simulink model "Vent_prop_valve_tuner"  (R2024b)
settings: Solver=ode15s  StartTime=0.0  StopTime=300  RelTol=1e-3
settings Model: Creator=MW  LastModifiedBy=MW

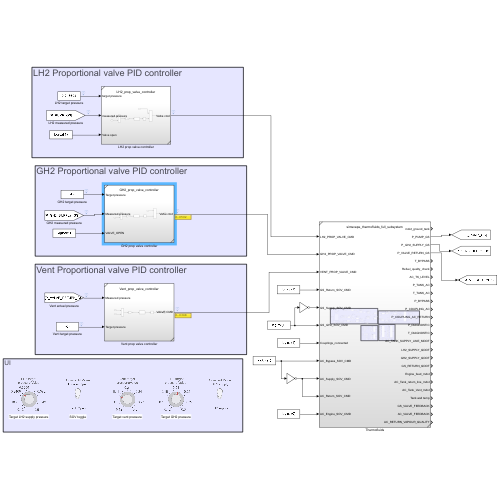
[thumbnail: Simulink's stored preview of the top-level diagram]
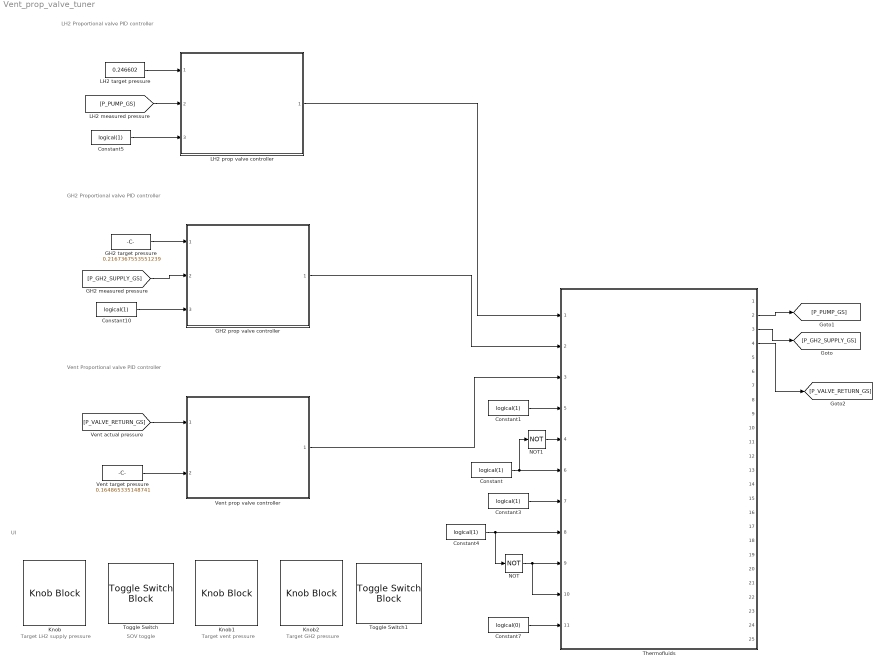
== system Vent_prop_valve_tuner ==
  note: Target LH2 supply pressure
  note: UI
  note: GH2 Proportional valve PID controller
  note: Target vent pressure
  note: SOV toggle
  note: LH2 Proportional valve PID controller
  note: Vent Proportional valve PID controller
  note: Target GH2 pressure
  Constant{,1,3..5,10} (6 alike) : Constant  Value=logical(1)
  Constant7 : Constant  Value=logical(0)
  GH2 prop valve controller : Subsystem  ReferencedSubsystem=GH2_prop_valve_controller
  GH2 target pressure : Constant  Value=0.2167367553551239
  Knob : KnobBlock  ScaleMin=0.12  ScaleMax=0.5
  Knob1 : KnobBlock  ScaleMin=0.12  ScaleMax=0.3
  Knob2 : KnobBlock  ScaleMin=0.12  ScaleMax=0.3
  LH2 prop valve controller : Subsystem  ReferencedSubsystem=LH2_prop_valve_controller
  LH2 target pressure : Constant  Value=0.246602
  NOT : Logic  Operator=NOT  IconShape=distinctive  AllPortsSameDT=off  OutDataTypeStr=boolean
  NOT1 : Logic  Operator=NOT  IconShape=distinctive  AllPortsSameDT=off  OutDataTypeStr=boolean
  Thermofluids : Subsystem  ReferencedSubsystem=simscape_thermofluids_full_subsystem
      settings: PortSchema="{\"entries\":[{\"content\":{\"sides\":[{\"content\":{\"connectorIds\":[\"In1\",\"In2\",\"In3\",\"In5\",\"In4\",\"In6\",\"In7\",\"In8\",\"In9\",\"In10\",\"In11\"]},\"type\":\"ConnectorPlacement.EquallySpacedRectSide\",\"uuid\":\"0abe1c09-fd1c-4f21-adb2-1ba1f178e40f\"},{\"content\":{\"connectorIds\":[\"Out1\",\"Out2\",\"Out3\",\"Out4\",\"Out5\",\"Out6\",\"Out7\",\"Out8\",\"Out9\",\"Out10\",\"Out11\",\"Out12\",\"Out13\",\"Out14\",\"Out15\",\"Out16\",\"Out17\",\"Out18\",\"Out19\",\"Out20\",\"Out21\",\"Out22\",\"Out23\",\"Out24\",\"Out25\"],\"side\":\"RIGHT\"},\"type\":\"ConnectorPlacement.EquallySpacedRectSide\",\"uuid\":\"d1a7e852-e313-42b4-9b52-713a379b8745\"},{\"content\":{\"side\":\"TOP\"},\"type\":\"ConnectorPlacement.EquallySpacedRectSide\",\"uuid\":\"bcf0416b-035c-45e3-b36d-7b1188a80ffd\"}]},\"type\":\"ConnectorPlacement.EquallySpacedConnector\",\"uuid\":\"eb213e55-2670-4e0e-a421-e9d6b5e6eb19\"}],\"packageUris\":[\"http://schema.mathworks.com/mf0/Connector/R2020b\"],\"version\":\"1.0\"}"
  Toggle Switch : ToggleSwitchBlock
      settings: Values={{'Tank Open', 'Bypass Open'}, [0 1]}
  Toggle Switch1 : ToggleSwitchBlock
      settings: Values={{'LH2 supply', 'GH2 supply'}, [0 1]}
  Vent prop valve controller : Subsystem  ReferencedSubsystem=Vent_prop_valve_controller
  Vent target pressure : Constant  Value=0.164865335148741
  wires:
  Constant1/1 -> Thermofluids/5
  Constant3/1 -> Thermofluids/7
  Constant4/1 -> NOT/1, Thermofluids/8
  NOT/1 -> Thermofluids/9, Thermofluids/10
  Constant7/1 -> Thermofluids/11
  GH2 target pressure/1 -> GH2 prop valve controller/1
  Constant10/1 -> GH2 prop valve controller/3
  [P_GH2_SUPPLY_GS] -> GH2 prop valve controller/2
  Thermofluids/3 -> [P_GH2_SUPPLY_GS]
  LH2 prop valve controller/1 -> Thermofluids/1
  GH2 prop valve controller/1 -> Thermofluids/2
  LH2 target pressure/1 -> LH2 prop valve controller/1
  [P_PUMP_GS] -> LH2 prop valve controller/2
  Constant5/1 -> LH2 prop valve controller/3
  Thermofluids/2 -> [P_PUMP_GS]
  Vent prop valve controller/1 -> Thermofluids/3
  Vent target pressure/1 -> Vent prop valve controller/2
  Thermofluids/4 -> [P_VALVE_RETURN_GS]
  [P_VALVE_RETURN_GS] -> Vent prop valve controller/1
  NOT1/1 -> Thermofluids/4
  Constant/1 -> Thermofluids/6, NOT1/1
